simulink model "youbot_motor_joint3"  (R2017b)
settings: Solver=VariableStepAuto  StartTime=0.0  StopTime=5  RelTol=1e-3
values from neighbouring files (symbols this model uses):
  B_env = 1.8    [motor_model_kuka_youbot.m]    (also in motor_model_kuka_youbot2.m = 0.01)
  I_env = 0.1    [motor_model_kuka_youbot.m]
  J = Jm + 1/(N^2)*(Jr + Jch)    (= 1.2077288055e-05)    [motor_model_kuka_youbot.m]    (also in motor_model_kuka_youbot2.m = 0.000181)
  K = k    (= 10)    [motor_model_kuka_youbot.m]    (also in motor_model_kuka_youbot2.m = i/1000)
  K_cur = Ki    (= 3.54813389234)    [Untitled.m]    (also in motor_model_kuka_youbot.m = 3000; motor_model_kuka_youbot2.m = 11.71875)
  K_env = 25    [motor_model_kuka_youbot.m]    (also in motor_model_kuka_youbot2.m = 1)
  K_pos = 200/256    (= 0.78125)    [motor_model_kuka_youbot.m]
  Ke = 51.1e-3    (= 0.0511)    [motor_model_kuka_youbot.m]    (also in motor_model_kuka_youbot2.m = 1.10867309417)
  kf = R*Jm/L * 1e-6    (= 1.85e-11)    [motor_model_kuka_youbot.m]    (also in motor_model_kuka_youbot2.m = 0.000237684665227)
  Ki = 10^(11/20)    (= 3.54813389234)    [Untitled.m]    (also in motor_model_kuka_youbot.m = 1; motor_model_kuka_youbot2.m = j/1000)
  Ki_cur = Ki/Ti    (= 17740.6694617)    [Untitled.m]    (also in motor_model_kuka_youbot.m = 3000; motor_model_kuka_youbot2.m = 0.0114440917969)
  Kt = 51e-3    (= 0.051)    [motor_model_kuka_youbot.m]    (also in motor_model_kuka_youbot2.m = 0.0369)
  Kv = 200    [motor_model_kuka_youbot.m]    (also in motor_model_kuka_youbot2.m = 0.78125)
  Kvi = 1000/65536    (= 0.0152587890625)    [motor_model_kuka_youbot.m]
  L = 2.24    [motor_model_kuka_youbot.m]    (also in motor_model_kuka_youbot2.m = 0.000463)
  N = 71    [motor_model_kuka_youbot.m]    (also in motor_model_kuka_youbot2.m = 10)
  R = 4.48    [motor_model_kuka_youbot.m]    (also in motor_model_kuka_youbot2.m = 0.608)
  weight = m*[0;0;-g]    [motor_model_kuka_youbot.m]
undefined symbols (not defined in the file or in its folder): Ki_pos
libraries: simulink x6, vrlib x1
settings Model: Creator=fortineau_vin  LastModifiedBy=fortineau_vin

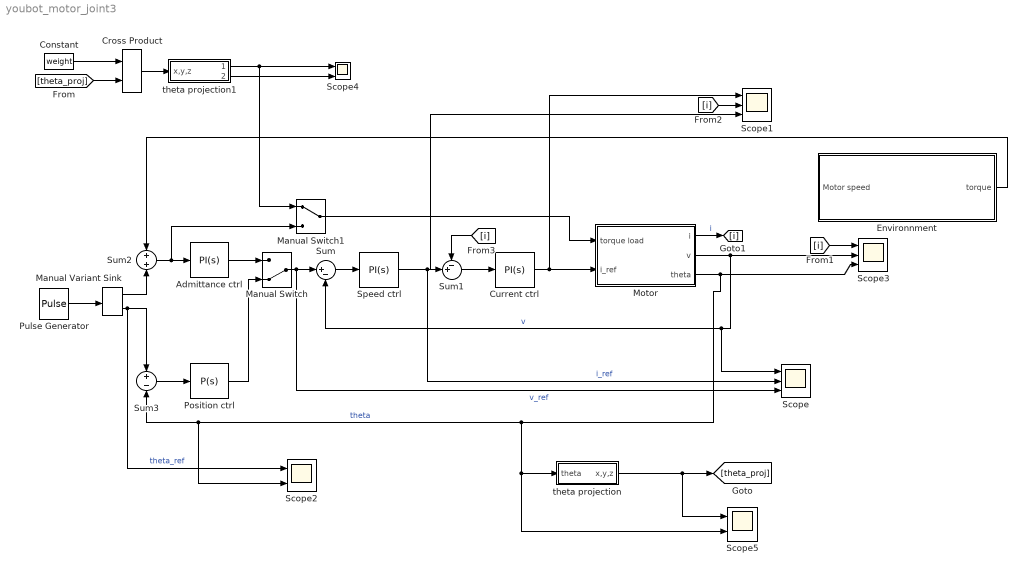
== system youbot_motor_joint3 ==
  Admittance ctrl : simulink/Continuous/PID Controller  Controller=PI  TimeDomain=Continuous-time  SampleTime=-1  IntegratorMethod=Forward Euler  FilterMethod=Forward Euler  Form=Parallel  UseFilter=on  ControllerParametersSource=internal  P=K  I=Ki  D=0  N=100  InitialConditionSource=internal  InitialConditionForIntegrator=0  InitialConditionForFilter=0  ExternalReset=none  LimitOutput=off  UpperSaturationLimit=inf  LowerSaturationLimit=-inf  LinearizeAsGain=on  AntiWindupMode=none  Kb=1  TrackingMode=off  Kt=1  PParamMin=[]  PParamMax=[]  IParamMin=[]  IParamMax=[]  DParamMin=[]  DParamMax=[]  NParamMin=[]  NParamMax=[]  KbParamMin=[]  KbParamMax=[]  KtParamMin=[]  KtParamMax=[]  POutMin=[]  POutMax=[]  IOutMin=[]  IOutMax=[]  DOutMin=[]  DOutMax=[]  NOutMin=[]  NOutMax=[]  KbOutMin=[]  KbOutMax=[]  KtOutMin=[]  KtOutMax=[]  IntegratorOutMin=[]  IntegratorOutMax=[]  FilterOutMin=[]  FilterOutMax=[]  SumOutMin=[]  SumOutMax=[]  SumI1OutMin=[]  SumI1OutMax=[]  SumI2OutMin=[]  SumI2OutMax=[]  SumI3OutMin=[]  SumI3OutMax=[]  SumDOutMin=[]  SumDOutMax=[]  SaturationOutMin=[]  SaturationOutMax=[]  IntegratorContinuousStateAttributes=''  IntegratorStateMustResolveToSignalObject=off  IntegratorRTWStateStorageClass=Auto  FilterContinuousStateAttributes=''  FilterStateMustResolveToSignalObject=off  FilterRTWStateStorageClass=Auto  DifferentiatorICPrevScaledInput=0  DifferentiatorOutMin=[]  DifferentiatorOutMax=[]  InitialConditionSetting=State (most efficient)  FilterDiffOutCoefMin=[]  FilterDiffOutCoefMax=[]  SumDenOutMin=[]  SumDenOutMax=[]  SumNumOutMin=[]  SumNumOutMax=[]  ReciprocalOutMin=[]  ReciprocalOutMax=[]  DivideOutMin=[]  DivideOutMax=[]  TunerSelectOption=Transfer Function Based (PID Tuner App)
  Constant : Constant  Value=weight
  Cross Product : vrlib/Utilities/Cross Product
      settings: SourceProductBaseCode=VR
  Current ctrl : simulink/Continuous/PID Controller  Controller=PI  TimeDomain=Continuous-time  SampleTime=-1  IntegratorMethod=Forward Euler  FilterMethod=Forward Euler  Form=Parallel  UseFilter=on  ControllerParametersSource=internal  P=K_cur  I=Ki_cur  D=0  N=100  InitialConditionSource=internal  InitialConditionForIntegrator=0  InitialConditionForFilter=0  ExternalReset=none  LimitOutput=off  UpperSaturationLimit=inf  LowerSaturationLimit=-inf  LinearizeAsGain=on  AntiWindupMode=none  Kb=1  TrackingMode=off  Kt=1  PParamMin=[]  PParamMax=[]  IParamMin=[]  IParamMax=[]  DParamMin=[]  DParamMax=[]  NParamMin=[]  NParamMax=[]  KbParamMin=[]  KbParamMax=[]  KtParamMin=[]  KtParamMax=[]  POutMin=[]  POutMax=[]  IOutMin=[]  IOutMax=[]  DOutMin=[]  DOutMax=[]  NOutMin=[]  NOutMax=[]  KbOutMin=[]  KbOutMax=[]  KtOutMin=[]  KtOutMax=[]  IntegratorOutMin=[]  IntegratorOutMax=[]  FilterOutMin=[]  FilterOutMax=[]  SumOutMin=[]  SumOutMax=[]  SumI1OutMin=[]  SumI1OutMax=[]  SumI2OutMin=[]  SumI2OutMax=[]  SumI3OutMin=[]  SumI3OutMax=[]  SumDOutMin=[]  SumDOutMax=[]  SaturationOutMin=[]  SaturationOutMax=[]  IntegratorContinuousStateAttributes=''  IntegratorStateMustResolveToSignalObject=off  IntegratorRTWStateStorageClass=Auto  FilterContinuousStateAttributes=''  FilterStateMustResolveToSignalObject=off  FilterRTWStateStorageClass=Auto  DifferentiatorICPrevScaledInput=0  DifferentiatorOutMin=[]  DifferentiatorOutMax=[]  InitialConditionSetting=State (most efficient)  FilterDiffOutCoefMin=[]  FilterDiffOutCoefMax=[]  SumDenOutMin=[]  SumDenOutMax=[]  SumNumOutMin=[]  SumNumOutMax=[]  ReciprocalOutMin=[]  ReciprocalOutMax=[]  DivideOutMin=[]  DivideOutMax=[]  TunerSelectOption=Transfer Function Based (PID Tuner App)
  "Environnment " : Subsystem
  Manual Variant Sink : simulink/Signal Routing/Manual Variant Sink  NumChoices=2  OverrideUsingVariant=V_2
      settings: SourceProductName=Simulink
  Manual Switch : ManualSwitch  CurrentSetting=0
  Manual Switch1 : ManualSwitch
  Motor : Subsystem
  Position ctrl : simulink/Continuous/PID Controller  Controller=P  TimeDomain=Continuous-time  SampleTime=-1  IntegratorMethod=Forward Euler  FilterMethod=Forward Euler  Form=Parallel  UseFilter=on  ControllerParametersSource=internal  P=K_pos  I=Ki_pos  D=0  N=100  InitialConditionSource=internal  InitialConditionForIntegrator=0  InitialConditionForFilter=0  ExternalReset=none  LimitOutput=off  UpperSaturationLimit=inf  LowerSaturationLimit=-inf  LinearizeAsGain=on  AntiWindupMode=none  Kb=1  TrackingMode=off  Kt=1  PParamMin=[]  PParamMax=[]  IParamMin=[]  IParamMax=[]  DParamMin=[]  DParamMax=[]  NParamMin=[]  NParamMax=[]  KbParamMin=[]  KbParamMax=[]  KtParamMin=[]  KtParamMax=[]  POutMin=[]  POutMax=[]  IOutMin=[]  IOutMax=[]  DOutMin=[]  DOutMax=[]  NOutMin=[]  NOutMax=[]  KbOutMin=[]  KbOutMax=[]  KtOutMin=[]  KtOutMax=[]  IntegratorOutMin=[]  IntegratorOutMax=[]  FilterOutMin=[]  FilterOutMax=[]  SumOutMin=[]  SumOutMax=[]  SumI1OutMin=[]  SumI1OutMax=[]  SumI2OutMin=[]  SumI2OutMax=[]  SumI3OutMin=[]  SumI3OutMax=[]  SumDOutMin=[]  SumDOutMax=[]  SaturationOutMin=[]  SaturationOutMax=[]  IntegratorContinuousStateAttributes=''  IntegratorStateMustResolveToSignalObject=off  IntegratorRTWStateStorageClass=Auto  FilterContinuousStateAttributes=''  FilterStateMustResolveToSignalObject=off  FilterRTWStateStorageClass=Auto  DifferentiatorICPrevScaledInput=0  DifferentiatorOutMin=[]  DifferentiatorOutMax=[]  InitialConditionSetting=State (most efficient)  FilterDiffOutCoefMin=[]  FilterDiffOutCoefMax=[]  SumDenOutMin=[]  SumDenOutMax=[]  SumNumOutMin=[]  SumNumOutMax=[]  ReciprocalOutMin=[]  ReciprocalOutMax=[]  DivideOutMin=[]  DivideOutMax=[]  TunerSelectOption=Transfer Function Based (PID Tuner App)
  Pulse Generator : DiscretePulseGenerator  PulseType=Time based  Amplitude=90/180*pi  Period=10  PulseWidth=50
  Scope : Scope  NumInputPorts=3
  Scope1 : Scope  NumInputPorts=3
  Scope2 : Scope  NumInputPorts=2
  Scope3 : Scope  NumInputPorts=3
  Scope4 : Scope  NumInputPorts=2
  Scope5 : Scope  NumInputPorts=2
  Speed ctrl : simulink/Continuous/PID Controller  Controller=PI  TimeDomain=Continuous-time  SampleTime=-1  IntegratorMethod=Forward Euler  FilterMethod=Forward Euler  Form=Parallel  UseFilter=on  ControllerParametersSource=internal  P=Kv  I=Kvi  D=0  N=100  InitialConditionSource=internal  InitialConditionForIntegrator=0  InitialConditionForFilter=0  ExternalReset=none  LimitOutput=off  UpperSaturationLimit=inf  LowerSaturationLimit=-inf  LinearizeAsGain=on  AntiWindupMode=none  Kb=1  TrackingMode=off  Kt=1  PParamMin=[]  PParamMax=[]  IParamMin=[]  IParamMax=[]  DParamMin=[]  DParamMax=[]  NParamMin=[]  NParamMax=[]  KbParamMin=[]  KbParamMax=[]  KtParamMin=[]  KtParamMax=[]  POutMin=[]  POutMax=[]  IOutMin=[]  IOutMax=[]  DOutMin=[]  DOutMax=[]  NOutMin=[]  NOutMax=[]  KbOutMin=[]  KbOutMax=[]  KtOutMin=[]  KtOutMax=[]  IntegratorOutMin=[]  IntegratorOutMax=[]  FilterOutMin=[]  FilterOutMax=[]  SumOutMin=[]  SumOutMax=[]  SumI1OutMin=[]  SumI1OutMax=[]  SumI2OutMin=[]  SumI2OutMax=[]  SumI3OutMin=[]  SumI3OutMax=[]  SumDOutMin=[]  SumDOutMax=[]  SaturationOutMin=[]  SaturationOutMax=[]  IntegratorContinuousStateAttributes=''  IntegratorStateMustResolveToSignalObject=off  IntegratorRTWStateStorageClass=Auto  FilterContinuousStateAttributes=''  FilterStateMustResolveToSignalObject=off  FilterRTWStateStorageClass=Auto  DifferentiatorICPrevScaledInput=0  DifferentiatorOutMin=[]  DifferentiatorOutMax=[]  InitialConditionSetting=State (most efficient)  FilterDiffOutCoefMin=[]  FilterDiffOutCoefMax=[]  SumDenOutMin=[]  SumDenOutMax=[]  SumNumOutMin=[]  SumNumOutMax=[]  ReciprocalOutMin=[]  ReciprocalOutMax=[]  DivideOutMin=[]  DivideOutMax=[]  TunerSelectOption=Transfer Function Based (PID Tuner App)
  Sum : Sum  Inputs=|+-
  Sum1 : Sum  Inputs=-+|
  Sum2 : Sum  Inputs=+|+
  Sum3 : Sum  Inputs=+|-
  theta projection : Subsystem
  theta projection1 : Subsystem
  wires:
  Sum1/1 -> Current ctrl/1
  Speed ctrl/1 -> Scope/2, Scope1/3, Sum1/2  "i_ref"
  Motor/2(v) -> Scope3/2, Scope/1, Sum/2  "v"
  "Environnment "/1(torque) -> Sum2/1
  Pulse Generator/1 -> Manual Variant Sink/1
  Sum/1 -> Speed ctrl/1
  Admittance ctrl/1 -> Manual Switch/1
  Manual Switch/1 -> Scope/3, Sum/1  "v_ref"
  Position ctrl/1 -> Manual Switch/2
  Sum3/1 -> Position ctrl/1
  Motor/3(theta) -> Scope3/3, Scope2/2, Sum3/2, theta projection/1(theta), Scope5/2  "theta"
  Current ctrl/1 -> Motor/2(i_ref), Scope1/1
  Manual Variant Sink/1 -> Sum2/2
  Manual Variant Sink/2 -> Scope2/1, Sum3/1  "theta_ref"
  Manual Switch1/1 -> Motor/1(torque load)
  Sum2/1 -> Manual Switch1/2, Admittance ctrl/1
  Constant/1 -> Cross Product/1
  [theta_proj] -> Cross Product/2
  theta projection/1(x,y,z) -> Scope5/1, [theta_proj]
  Cross Product/1 -> theta projection1/1(x,y,z)
  theta projection1/1(T_pert 1) -> Manual Switch1/1, Scope4/1
  theta projection1/2(T_pert 2) -> Scope4/2
  Motor/1(i) -> [i]  "i"
  [i] -> Scope3/1
  [i] -> Scope1/2
  [i] -> Sum1/1

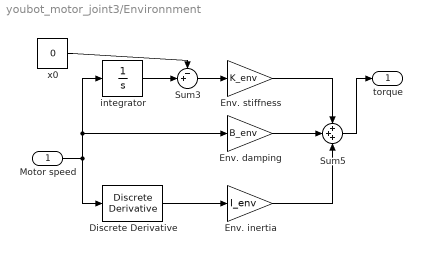
== system youbot_motor_joint3/Environnment  ==
  Motor speed : Inport
  Discrete Derivative : simulink/Discrete/Discrete Derivative  gainval=1.0  ICPrevScaledInput=0.0  OutMin=[]  OutMax=[]  OutDataType=fixdt(1, 16)  OutScaling=2^-10  DoSatur=off
  Env. damping : Gain  Gain=B_env
  Env. inertia : Gain  Gain=I_env
  Env. stiffness : Gain  Gain=K_env
  Sum3 : Sum  Inputs=-+|
  Sum5 : Sum  Inputs=+++
  integrator : TransferFcn  Denominator=[1 0]
  x0 : Constant  Value=0
  torque : Outport
  wires:
  Env. damping/1 -> Sum5/2
  Motor speed/1 -> Discrete Derivative/1, Env. damping/1, integrator/1
  Sum5/1 -> torque/1
  x0/1 -> Sum3/1
  integrator/1 -> Sum3/2
  Sum3/1 -> Env. stiffness/1
  Env. stiffness/1 -> Sum5/1
  Discrete Derivative/1 -> Env. inertia/1
  Env. inertia/1 -> Sum5/3

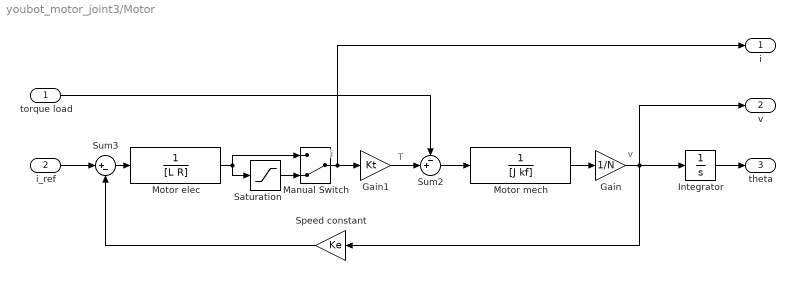
== system youbot_motor_joint3/Motor ==
  note: v
  note: T
  note: i
  torque load : Inport
  i_ref : Inport  Port=2
  Gain : Gain  Gain=1/N
  Gain1 : Gain  Gain=Kt
  Integrator : Integrator
  Manual Switch : ManualSwitch  CurrentSetting=0
  Motor elec : TransferFcn  Denominator=[L R]
  Motor mech : TransferFcn  Denominator=[J kf]
  Saturation : Saturate
  Speed constant : Gain  Gain=Ke
  Sum2 : Sum  Inputs=-+|
  Sum3 : Sum  Inputs=|+-
  i : Outport
  v : Outport  Port=2
  theta : Outport  Port=3
  wires:
  Manual Switch/1 -> i/1, Gain1/1
  Sum2/1 -> Motor mech/1
  Gain1/1 -> Sum2/2
  Gain/1 -> Integrator/1, v/1, Speed constant/1
  Motor mech/1 -> Gain/1
  torque load/1 -> Sum2/1
  Speed constant/1 -> Sum3/2
  Sum3/1 -> Motor elec/1
  i_ref/1 -> Sum3/1
  Saturation/1 -> Manual Switch/2
  Motor elec/1 -> Saturation/1, Manual Switch/1
  Integrator/1 -> theta/1

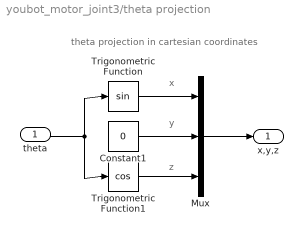
== system youbot_motor_joint3/theta projection ==
  note: z
  note: y
  note: x
  note: theta projection in cartesian coordinates
  theta : Inport
  Constant1 : Constant  Value=0
  Mux : Mux  Inputs=3
  Trigonometric Function : Trigonometry
  Trigonometric Function1 : Trigonometry  Operator=cos
  x,y,z : Outport
  wires:
  Constant1/1 -> Mux/2
  Trigonometric Function/1 -> Mux/1
  Trigonometric Function1/1 -> Mux/3
  Mux/1 -> x,y,z/1
  theta/1 -> Trigonometric Function/1, Trigonometric Function1/1

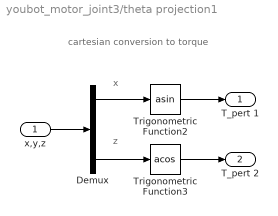
== system youbot_motor_joint3/theta projection1 ==
  note: z
  note: x
  note: cartesian conversion to torque
  x,y,z : Inport
  Demux : Demux  Outputs=3
  Trigonometric Function2 : Trigonometry  Operator=asin
  Trigonometric Function3 : Trigonometry  Operator=acos
  T_pert 1 : Outport
  T_pert 2 : Outport  Port=2
  wires:
  x,y,z/1 -> Demux/1
  Demux/1 -> Trigonometric Function2/1
  Demux/3 -> Trigonometric Function3/1
  Trigonometric Function2/1 -> T_pert 1/1
  Trigonometric Function3/1 -> T_pert 2/1
